simulink model "gm_sampleModel1618_sub"  (R2023a)
settings: Solver=VariableStepAuto  StartTime=0.0  StopTime=10.0  RelTol=1e-3
libraries: simulink x3, hdlsllib x2
settings Model: Creator=user1  LastModifiedBy=user1
settings OptimizationCC: BlockReduction=off  ConditionallyExecuteInputs=off
settings DebuggingCC: InheritedTsInSrcMsg=none

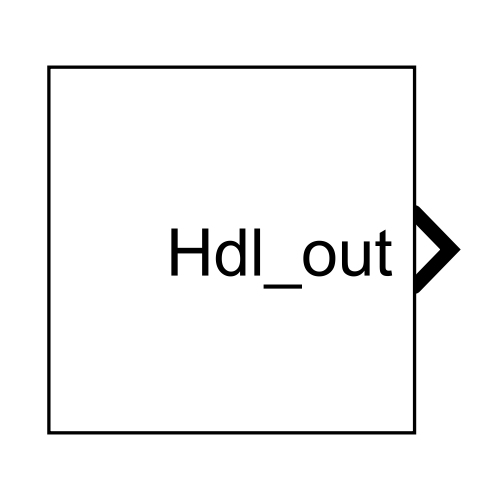
[thumbnail: Simulink's stored preview of the top-level diagram]
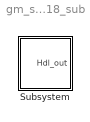
== system gm_sampleModel1618_sub ==
  Subsystem : Subsystem

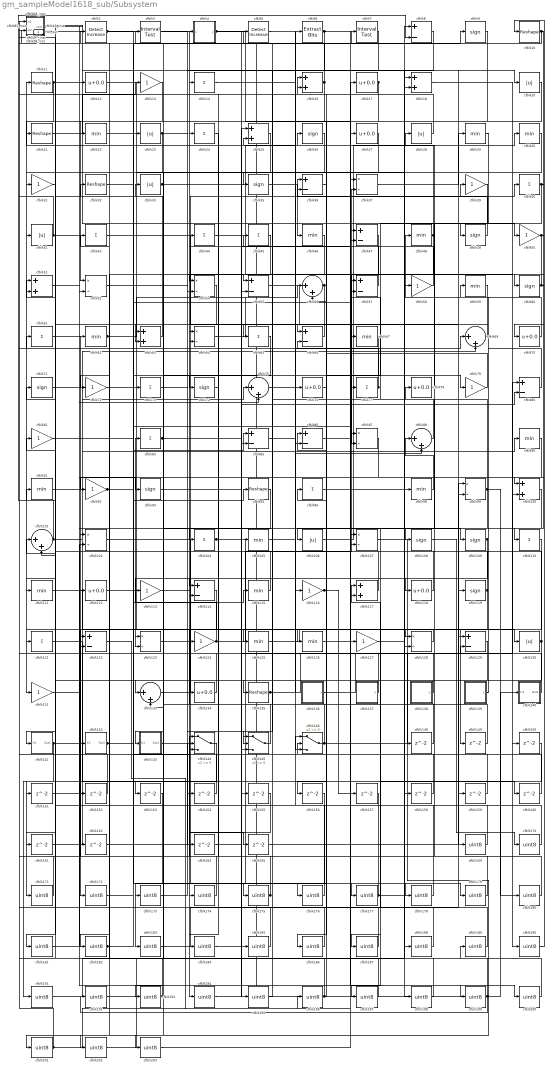
== system gm_sampleModel1618_sub/Subsystem ==
  cfblk1 : Constant  Value=0  OutDataTypeStr=uint8  SampleTime=1
  cfblk{10..11,21,32,95,135} (6 alike) : Reshape
  cfblk{16,18,25,51,63,100,117} (7 alike) : Sum  OutDataTypeStr=uint8
  cfblk{56,69,75,88,101,133} (6 alike) : Sum  Inputs=|++  OutDataTypeStr=uint8
  cfblk{37,52,54,64,87,99,102,107,123,128} (10 alike) : Product  Inputs=*/  OutDataTypeStr=uint8  RndMeth=Zero  SaturateOnIntegerOverflow=on
  cfblk{14,24,40,42,44..45,61,65,73,77,83,96,104,110,121} (15 alike) : Sum  Inputs=+  OutDataTypeStr=uint8
  cfblk{22,29..30,46,48,59,62,67,90..91,98,105,111,115,125..126} (16 alike) : MinMax  OutDataTypeStr=uint8
  cfblk{20,23,28,33,41,106,130} (7 alike) : Abs  OutDataTypeStr=uint8  SaturateOnIntegerOverflow=off
  cfblk{9,26,35,49,60,71,74,93,108..109,119} (11 alike) : Signum
  cfblk{12,17,27,70,76,78,112,118,134} (9 alike) : Bias  Bias=0.0  SaturateOnIntegerOverflow=off
  cfblk{13,31,39,50,58,72,79,81,92,113,116,124,127,131} (14 alike) : Gain  OutDataTypeStr=uint8
  cfblk{8,36,47,55,57,66,80,85..86,114,122,129} (12 alike) : Sum  Inputs=+-  OutDataTypeStr=uint8
  cfblk132_inst : Subsystem
  cfblk136 : Subsystem  mask(Counter Limited){uplimit=double(7), tsamp=double(-1)}
      mask prompts: uplimit "Simulink:masks:UpperLimit_MP"; tsamp "Simulink:masks:SampleTime_MP"
      mask help: Simulink:masks:CounterLimited_MD
      mask init:
      | nbits = double(8);
      | tsamp = double(-1);
      | uplimit = double(7);
  cfblk137 : Subsystem  mask(Counter Limited){uplimit=double(7), tsamp=double(-1)}
      mask prompts: uplimit "Simulink:masks:UpperLimit_MP"; tsamp "Simulink:masks:SampleTime_MP"
      mask help: Simulink:masks:CounterLimited_MD
      mask init:
      | nbits = double(8);
      | tsamp = double(-1);
      | uplimit = double(7);
  cfblk138 : Subsystem  mask(Counter Free-Running){NumBits=double(16), tsamp=double(-1)}
      mask prompts: NumBits "Simulink:masks:NumberOfBits_MP"; tsamp "Simulink:masks:SampleTime_MP"
      mask help: Simulink:masks:CounterFreeRunning_MD
  cfblk139 : Subsystem  mask(Counter Limited){uplimit=double(7), tsamp=double(-1)}
      mask prompts: uplimit "Simulink:masks:UpperLimit_MP"; tsamp "Simulink:masks:SampleTime_MP"
      mask help: Simulink:masks:CounterLimited_MD
      mask init:
      | nbits = double(8);
      | tsamp = double(-1);
      | uplimit = double(7);
  cfblk140 : Subsystem
  cfblk141 : Subsystem
  cfblk142 : Subsystem
  cfblk143 : Subsystem
  cfblk144 : Switch  OutDataTypeStr=uint8  SaturateOnIntegerOverflow=off  InputSameDT=off
  cfblk145 : Switch  OutDataTypeStr=uint8  SaturateOnIntegerOverflow=off  InputSameDT=off
  cfblk146 : Switch  OutDataTypeStr=uint8  SaturateOnIntegerOverflow=off  InputSameDT=off
  cfblk{148..162,164..165} (17 alike) : Delay  SampleTime=1
  cfblk15_inst : Subsystem
  cfblk{169..203} (35 alike) : DataTypeConversion  OutDataTypeStr=uint8  SaturateOnIntegerOverflow=off  RndMeth=Floor
  cfblk2 : simulink/Logic and Bit Operations/Detect Increase  vinit=0.0  OutDataTypeStr=uint8
      settings: LibrarySourceBlock=|
      | hdlsllib/Logic and Bit
      | Operations/Detect
      | Increase
  cfblk3 : hdlsllib/Logic and Bit Operations/Interval Test  IntervalClosedRight=on  uplimit=0.5  IntervalClosedLeft=on  lowlimit=-0.5  OutDataTypeStr=uint8
  cfblk34_inst : Subsystem
  cfblk38_inst : Subsystem
  cfblk4 : Subsystem  mask(Compare To Zero){relop=<=, OutDataTypeStr=uint8, ZeroCross=on}
      mask prompts: relop "Simulink:masks:Operator_MP"; OutDataTypeStr "Simulink:masks:OutputDataType_MP"; ZeroCross "Simulink:masks:EnableZerocrossingDetection_MP"
      mask help: Simulink:masks:CompareToZero_MD
      mask init:
      | OutDataTypeStr = 'uint8';
      | ZeroCross = 'on';
      | blkName = 'sampleModel1618_sub/Subsystem/cfblk4';
      | relop = '<=';
      | setValue = 'fixdt(0, 8)';
      mask TypeOptions relop: == | ~= | < | <= | >= | >
      mask TypeOptions OutDataTypeStr: Simulink:masks:uint8 | Simulink:masks:boolean
      mask Callback ZeroCross: sl('zeroCrossEnable', gcbh);
      mask Display: disp([relop,' 0'])
  cfblk43_inst : Subsystem
  cfblk5 : simulink/Logic and Bit Operations/Detect Increase  vinit=0.0  OutDataTypeStr=uint8
      settings: LibrarySourceBlock=|
      | hdlsllib/Logic and Bit
      | Operations/Detect
      | Increase
  cfblk6 : simulink/Logic and Bit Operations/Extract Bits  bitsToExtract=Upper half  numBits=8  bitIdxRange=[0 7]  outScalingMode=Preserve fixed-point scaling
      settings: LibrarySourceBlock=|
      | hdlsllib/Logic and Bit
      | Operations/Extract Bits
  cfblk68_inst : Subsystem
  cfblk7 : hdlsllib/Logic and Bit Operations/Interval Test  IntervalClosedRight=on  uplimit=0.5  IntervalClosedLeft=on  lowlimit=-0.5  OutDataTypeStr=uint8
  cfblk82_inst : Subsystem
  cfblk97_inst : Subsystem
  Hdl_out : Outport  OutDataTypeStr=uint8  SampleTime=1
  wires:
  cfblk1/1 -> cfblk50/1
  cfblk10/1 -> cfblk60/1, cfblk43_inst/2(in2)
  cfblk100/1 -> cfblk106/1
  cfblk101/1 -> cfblk8/2, cfblk109/1
  cfblk102/1 -> cfblk179/1
  cfblk104/1 -> cfblk178/1, cfblk105/1
  cfblk105/1 -> cfblk7/1
  cfblk106/1 -> cfblk30/1
  cfblk107/1 -> cfblk201/1
  cfblk108/1 -> cfblk170/1
  cfblk109/1 -> cfblk118/1, cfblk123/2
  cfblk11/1 -> cfblk12/1, cfblk131/1
  cfblk110/1 -> cfblk194/1
  cfblk111/1 -> cfblk130/1
  cfblk112/1 -> cfblk149/1
  cfblk113/1 -> cfblk175/1
  cfblk114/1 -> cfblk172/1
  cfblk115/1 -> cfblk61/1
  cfblk116/1 -> cfblk56/2, cfblk157/1, cfblk127/1
  cfblk117/1 -> cfblk71/1
  cfblk118/1 -> cfblk51/1
  cfblk119/1 -> cfblk38_inst/2(in2), cfblk143/1(In1)
  cfblk12/1 -> cfblk159/1
  cfblk121/1 -> cfblk153/1
  cfblk122/1 -> cfblk196/1
  cfblk123/1 -> cfblk4/1(u)
  cfblk124/1 -> cfblk37/2, cfblk83/1
  cfblk125/1 -> cfblk128/1
  cfblk126/1 -> cfblk37/1
  cfblk127/1 -> cfblk98/1
  cfblk128/1 -> cfblk121/1
  cfblk129/1 -> cfblk182/1
  cfblk13/1 -> cfblk52/1
  cfblk130/1 -> cfblk86/1, cfblk181/1
  cfblk131/1 -> cfblk62/1
  cfblk132_inst/1(out1) -> cfblk158/1
  cfblk133/1 -> cfblk39/1
  cfblk134/1 -> cfblk24/1
  cfblk135/1 -> cfblk76/1, cfblk99/1
  cfblk136/1(y) -> cfblk80/1
  cfblk137/1(y) -> cfblk132_inst/2(in2)
  cfblk138/1(y) -> cfblk8/1
  cfblk139/1(y) -> cfblk59/1
  cfblk14/1 -> cfblk116/1
  cfblk140/1(Out1) -> cfblk16/1
  cfblk141/1(Out1) -> cfblk191/1, cfblk90/1
  cfblk142/1(Out1) -> cfblk9/1, cfblk85/1
  cfblk143/1(Out1) -> cfblk165/1
  cfblk144/1 -> cfblk171/1
  cfblk145/1 -> cfblk97_inst/1(in1)
  cfblk146/1 -> cfblk100/2, cfblk64/1
  cfblk148/1 -> cfblk66/2
  cfblk149/1 -> cfblk114/2
  cfblk15_inst/1(out1) -> cfblk185/1
  cfblk150/1 -> cfblk197/1
  cfblk151/1 -> cfblk75/1
  cfblk152/1 -> cfblk51/2
  cfblk153/1 -> cfblk183/1
  cfblk154/1 -> cfblk101/1
  cfblk155/1 -> cfblk174/1
  cfblk156/1 -> cfblk173/1
  cfblk157/1 -> cfblk146/2
  cfblk158/1 -> cfblk64/2
  cfblk159/1 -> cfblk133/2
  cfblk16/1 -> cfblk135/1, cfblk3/1
  cfblk160/1 -> cfblk82_inst/1(in1)
  cfblk161/1 -> cfblk69/2
  cfblk162/1 -> cfblk195/1
  cfblk164/1 -> cfblk47/2
  cfblk165/1 -> cfblk119/1
  cfblk169/1 -> cfblk146/1
  cfblk17/1 -> cfblk85/2, cfblk156/1
  cfblk170/1 -> cfblk42/1
  cfblk171/1 -> cfblk82_inst/2(in2)
  cfblk172/1 -> cfblk144/1
  cfblk173/1 -> cfblk144/2
  cfblk174/1 -> cfblk144/3
  cfblk175/1 -> cfblk132_inst/1(in1), cfblk14/1
  cfblk176/1 -> cfblk113/1
  cfblk177/1 -> cfblk32/1, cfblk40/1
  cfblk178/1 -> cfblk81/1
  cfblk179/1 -> cfblk78/1
  cfblk18/1 -> cfblk190/1
  cfblk180/1 -> cfblk102/1
  cfblk181/1 -> cfblk102/2
  cfblk182/1 -> cfblk95/1, cfblk115/1
  cfblk183/1 -> cfblk129/1
  cfblk184/1 -> cfblk129/2
  cfblk185/1 -> cfblk152/1
  cfblk186/1 -> cfblk15_inst/1(in1)
  cfblk187/1 -> cfblk15_inst/2(in2)
  cfblk188/1 -> cfblk117/1
  cfblk189/1 -> cfblk96/1
  cfblk190/1 -> cfblk10/1
  cfblk191/1 -> cfblk18/1
  cfblk192/1 -> cfblk18/2
  cfblk193/1 -> cfblk43_inst/1(in1), cfblk142/1(In1)
  cfblk194/1 -> cfblk25/1
  cfblk195/1 -> cfblk25/2
  cfblk196/1 -> cfblk33/1, cfblk26/1
  cfblk197/1 -> cfblk122/1
  cfblk198/1 -> cfblk122/2
  cfblk199/1 -> cfblk192/1, cfblk189/1, Hdl_out/1, cfblk140/1(In1)
  cfblk2/1 -> cfblk86/2, cfblk125/1
  cfblk20/1 -> cfblk41/1
  cfblk200/1 -> cfblk91/1
  cfblk201/1 -> cfblk34_inst/1(in1), cfblk27/1
  cfblk202/1 -> cfblk107/1
  cfblk203/1 -> cfblk107/2
  cfblk21/1 -> cfblk13/1
  cfblk22/1 -> cfblk148/1
  cfblk23/1 -> cfblk55/1, cfblk31/1
  cfblk24/1 -> cfblk184/1
  cfblk25/1 -> cfblk193/1
  cfblk26/1 -> cfblk141/1(In1)
  cfblk27/1 -> cfblk114/1
  cfblk28/1 -> cfblk68_inst/1(in1)
  cfblk29/1 -> cfblk49/1
  cfblk3/1 -> cfblk145/2
  cfblk30/1 -> cfblk63/2
  cfblk31/1 -> cfblk111/1
  cfblk32/1 -> cfblk160/1
  cfblk33/1 -> cfblk6/1, cfblk87/2
  cfblk34_inst/1(out1) -> cfblk162/1
  cfblk35/1 -> cfblk46/1
  cfblk36/1 -> cfblk16/2
  cfblk37/1 -> cfblk29/1
  cfblk38_inst/1(out1) -> cfblk20/1, cfblk99/2
  cfblk39/1 -> cfblk108/1
  cfblk4/1(y) -> cfblk145/3, cfblk117/2
  cfblk40/1 -> cfblk70/1, cfblk67/1
  cfblk41/1 -> cfblk93/1, cfblk34_inst/2(in2)
  cfblk42/1 -> cfblk169/1
  cfblk43_inst/1(out1) -> cfblk52/2, cfblk73/1
  cfblk44/1 -> cfblk150/1
  cfblk45/1 -> cfblk72/1
  cfblk46/1 -> cfblk202/1
  cfblk47/1 -> cfblk55/2
  cfblk48/1 -> cfblk11/1, cfblk126/1
  cfblk49/1 -> cfblk36/1
  cfblk5/1 -> cfblk128/2
  cfblk50/1 -> cfblk146/3, cfblk110/1
  cfblk51/1 -> cfblk75/2
  cfblk52/1 -> cfblk134/1
  cfblk54/1 -> cfblk161/1
  cfblk55/1 -> cfblk198/1
  cfblk56/1 -> cfblk74/1, cfblk151/1
  cfblk57/1 -> cfblk44/1
  cfblk58/1 -> cfblk45/1
  cfblk59/1 -> cfblk77/1
  cfblk6/1 -> cfblk35/1, cfblk200/1
  cfblk60/1 -> cfblk100/1, cfblk54/1
  cfblk61/1 -> cfblk104/1
  cfblk62/1 -> cfblk56/1, cfblk79/1
  cfblk63/1 -> cfblk21/1
  cfblk64/1 -> cfblk47/1
  cfblk65/1 -> cfblk133/1
  cfblk66/1 -> cfblk63/1
  cfblk67/1 -> cfblk176/1
  cfblk68_inst/1(out1) -> cfblk154/1
  cfblk69/1 -> cfblk66/1
  cfblk7/1 -> cfblk54/2
  cfblk70/1 -> cfblk48/1
  cfblk71/1 -> cfblk112/1
  cfblk72/1 -> cfblk23/1
  cfblk73/1 -> cfblk164/1
  cfblk74/1 -> cfblk124/1
  cfblk75/1 -> cfblk69/1
  cfblk76/1 -> cfblk186/1
  cfblk77/1 -> cfblk97_inst/2(in2), cfblk68_inst/2(in2), cfblk38_inst/1(in1)
  cfblk78/1 -> cfblk28/1
  cfblk79/1 -> cfblk36/2
  cfblk8/1 -> cfblk145/1
  cfblk80/1 -> cfblk58/1
  cfblk81/1 -> cfblk177/1
  cfblk82_inst/1(out1) -> cfblk101/2
  cfblk83/1 -> cfblk87/1, cfblk155/1
  cfblk85/1 -> cfblk88/2
  cfblk86/1 -> cfblk17/1
  cfblk87/1 -> cfblk92/1
  cfblk88/1 -> cfblk57/1
  cfblk9/1 -> cfblk65/1
  cfblk90/1 -> cfblk203/1
  cfblk91/1 -> cfblk199/1
  cfblk92/1 -> cfblk57/2, cfblk2/1
  cfblk93/1 -> cfblk80/2
  cfblk95/1 -> cfblk123/1
  cfblk96/1 -> cfblk188/1
  cfblk97_inst/1(out1) -> cfblk22/1
  cfblk98/1 -> cfblk88/1
  cfblk99/1 -> cfblk187/1, cfblk180/1, cfblk5/1

== system gm_sampleModel1618_sub/Subsystem/cfblk132_inst ==
  in1 : Inport  OutDataTypeStr=uint8  SampleTime=1
  in2 : Inport  Port=2  OutDataTypeStr=uint8  SampleTime=1
  mul_cfblk132_dotp_mulcomp : Product  Inputs=**  OutDataTypeStr=uint8  SampleTime=1
  out1 : Outport  OutDataTypeStr=uint8  SampleTime=1
  wires:
  in1/1 -> mul_cfblk132_dotp_mulcomp/1
  in2/1 -> mul_cfblk132_dotp_mulcomp/2
  mul_cfblk132_dotp_mulcomp/1 -> out1/1

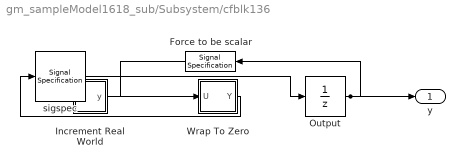
== system gm_sampleModel1618_sub/Subsystem/cfblk136 ==
  Force to be scalar : SignalSpecification  DisableCoverage=on  Dimensions=1
  Increment Real World : Subsystem  mask(Real World Value Increment){}
      mask help: Simulink:masks:RealWorldValueIncrement_MD
      mask Display: disp('V++')
  Output : UnitDelay  InitialCondition=0.0  SampleTime=tsamp  HasFrameUpgradeWarning=on
  Wrap To Zero : Subsystem  mask(Wrap To Zero){Threshold=double(7)}
      mask prompts: Threshold "Simulink:masks:Threshold_MP"
      mask help: Simulink:masks:WrapToZero_MD
  sigspec : SignalSpecification  OutDataTypeStr=uint8  Dimensions=1
  y : Outport  SampleTime=1
  wires:
  Force to be scalar/1 -> Increment Real World/1(u)
  Increment Real World/1(y) -> Wrap To Zero/1(U)
  Output/1 -> Force to be scalar/1, y/1
  Wrap To Zero/1(Y) -> sigspec/1
  sigspec/1 -> Output/1

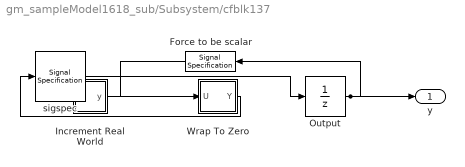
== system gm_sampleModel1618_sub/Subsystem/cfblk137 ==
  Force to be scalar : SignalSpecification  DisableCoverage=on  Dimensions=1
  Increment Real World : Subsystem  mask(Real World Value Increment){}
      mask help: Simulink:masks:RealWorldValueIncrement_MD
      mask Display: disp('V++')
  Output : UnitDelay  InitialCondition=0.0  SampleTime=tsamp  HasFrameUpgradeWarning=on
  Wrap To Zero : Subsystem  mask(Wrap To Zero){Threshold=double(7)}
      mask prompts: Threshold "Simulink:masks:Threshold_MP"
      mask help: Simulink:masks:WrapToZero_MD
  sigspec : SignalSpecification  OutDataTypeStr=uint8  Dimensions=1
  y : Outport  SampleTime=1
  wires:
  Force to be scalar/1 -> Increment Real World/1(u)
  Increment Real World/1(y) -> Wrap To Zero/1(U)
  Output/1 -> Force to be scalar/1, y/1
  Wrap To Zero/1(Y) -> sigspec/1
  sigspec/1 -> Output/1

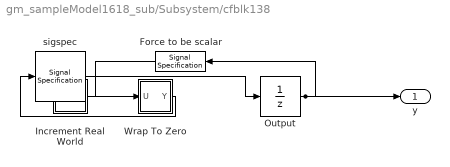
== system gm_sampleModel1618_sub/Subsystem/cfblk138 ==
  Force to be scalar : SignalSpecification  DisableCoverage=on  Dimensions=1
  Increment Real World : Subsystem  mask(Real World Value Increment){}
      mask help: Simulink:masks:RealWorldValueIncrement_MD
      mask Display: disp('V++')
  Output : UnitDelay  InitialCondition=0.0  SampleTime=tsamp  HasFrameUpgradeWarning=on
  Wrap To Zero : Subsystem  mask(Wrap To Zero){Threshold=double(65535)}
      mask prompts: Threshold "Simulink:masks:Threshold_MP"
      mask help: Simulink:masks:WrapToZero_MD
  sigspec : SignalSpecification  OutDataTypeStr=uint16  Dimensions=1
  y : Outport  SampleTime=1
  wires:
  Force to be scalar/1 -> Increment Real World/1(u)
  Increment Real World/1(y) -> Wrap To Zero/1(U)
  Output/1 -> Force to be scalar/1, y/1
  Wrap To Zero/1(Y) -> sigspec/1
  sigspec/1 -> Output/1

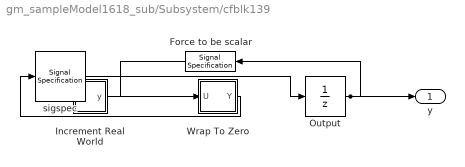
== system gm_sampleModel1618_sub/Subsystem/cfblk139 ==
  Force to be scalar : SignalSpecification  DisableCoverage=on  Dimensions=1
  Increment Real World : Subsystem  mask(Real World Value Increment){}
      mask help: Simulink:masks:RealWorldValueIncrement_MD
      mask Display: disp('V++')
  Output : UnitDelay  InitialCondition=0.0  SampleTime=tsamp  HasFrameUpgradeWarning=on
  Wrap To Zero : Subsystem  mask(Wrap To Zero){Threshold=double(7)}
      mask prompts: Threshold "Simulink:masks:Threshold_MP"
      mask help: Simulink:masks:WrapToZero_MD
  sigspec : SignalSpecification  OutDataTypeStr=uint8  Dimensions=1
  y : Outport  SampleTime=1
  wires:
  Force to be scalar/1 -> Increment Real World/1(u)
  Increment Real World/1(y) -> Wrap To Zero/1(U)
  Output/1 -> Force to be scalar/1, y/1
  Wrap To Zero/1(Y) -> sigspec/1
  sigspec/1 -> Output/1

== system gm_sampleModel1618_sub/Subsystem/cfblk140 ==
  In1 : Inport  OutDataTypeStr=uint8  PortDimensions=1  SampleTime=1
  Out1 : Outport  SampleTime=1
  wires:
  In1/1 -> Out1/1

== system gm_sampleModel1618_sub/Subsystem/cfblk141 ==
  In1 : Inport  OutDataTypeStr=uint8  PortDimensions=1  SampleTime=1
  Out1 : Outport  SampleTime=1
  wires:
  In1/1 -> Out1/1

== system gm_sampleModel1618_sub/Subsystem/cfblk142 ==
  In1 : Inport  OutDataTypeStr=uint8  PortDimensions=1  SampleTime=1
  Out1 : Outport  SampleTime=1
  wires:
  In1/1 -> Out1/1

== system gm_sampleModel1618_sub/Subsystem/cfblk143 ==
  In1 : Inport  OutDataTypeStr=uint8  PortDimensions=1  SampleTime=1
  Out1 : Outport  SampleTime=1
  wires:
  In1/1 -> Out1/1

== system gm_sampleModel1618_sub/Subsystem/cfblk15_inst ==
  in1 : Inport  OutDataTypeStr=uint8  SampleTime=1
  in2 : Inport  Port=2  OutDataTypeStr=uint8  SampleTime=1
  mul_cfblk15_dotp_mulcomp : Product  Inputs=**  OutDataTypeStr=uint8  SampleTime=1
  out1 : Outport  OutDataTypeStr=uint8  SampleTime=1
  wires:
  in1/1 -> mul_cfblk15_dotp_mulcomp/1
  in2/1 -> mul_cfblk15_dotp_mulcomp/2
  mul_cfblk15_dotp_mulcomp/1 -> out1/1

== system gm_sampleModel1618_sub/Subsystem/cfblk34_inst ==
  in1 : Inport  OutDataTypeStr=uint8  SampleTime=1
  in2 : Inport  Port=2  OutDataTypeStr=uint8  SampleTime=1
  mul_cfblk34_dotp_mulcomp : Product  Inputs=**  OutDataTypeStr=uint8  SampleTime=1
  out1 : Outport  OutDataTypeStr=uint8  SampleTime=1
  wires:
  in1/1 -> mul_cfblk34_dotp_mulcomp/1
  in2/1 -> mul_cfblk34_dotp_mulcomp/2
  mul_cfblk34_dotp_mulcomp/1 -> out1/1

== system gm_sampleModel1618_sub/Subsystem/cfblk38_inst ==
  in1 : Inport  OutDataTypeStr=uint8  SampleTime=1
  in2 : Inport  Port=2  OutDataTypeStr=uint8  SampleTime=1
  mul_cfblk38_dotp_mulcomp : Product  Inputs=**  OutDataTypeStr=uint8  SampleTime=1
  out1 : Outport  OutDataTypeStr=uint8  SampleTime=1
  wires:
  in1/1 -> mul_cfblk38_dotp_mulcomp/1
  in2/1 -> mul_cfblk38_dotp_mulcomp/2
  mul_cfblk38_dotp_mulcomp/1 -> out1/1

== system gm_sampleModel1618_sub/Subsystem/cfblk4 ==
  u : Inport  OutDataTypeStr=uint8  SampleTime=1
  Compare : RelationalOperator  Operator=<=  OutDataTypeStr=fixdt(0, 8)
  Constant : Constant  DisableCoverage=on  Value=0  OutDataTypeStr=Inherit: Inherit via back propagation  SampleTime=-1  PreserveConstantTs=on
  y : Outport  SampleTime=1
  wires:
  u/1 -> Compare/1
  Compare/1 -> y/1
  Constant/1 -> Compare/2

== system gm_sampleModel1618_sub/Subsystem/cfblk43_inst ==
  in1 : Inport  OutDataTypeStr=uint8  SampleTime=1
  in2 : Inport  Port=2  OutDataTypeStr=uint8  SampleTime=1
  mul_cfblk43_dotp_mulcomp : Product  Inputs=**  OutDataTypeStr=uint8  SampleTime=1
  out1 : Outport  OutDataTypeStr=uint8  SampleTime=1
  wires:
  in1/1 -> mul_cfblk43_dotp_mulcomp/1
  in2/1 -> mul_cfblk43_dotp_mulcomp/2
  mul_cfblk43_dotp_mulcomp/1 -> out1/1

== system gm_sampleModel1618_sub/Subsystem/cfblk68_inst ==
  in1 : Inport  OutDataTypeStr=uint8  SampleTime=1
  in2 : Inport  Port=2  OutDataTypeStr=uint8  SampleTime=1
  mul_cfblk68_dotp_mulcomp : Product  Inputs=**  OutDataTypeStr=uint8  SampleTime=1
  out1 : Outport  OutDataTypeStr=uint8  SampleTime=1
  wires:
  in1/1 -> mul_cfblk68_dotp_mulcomp/1
  in2/1 -> mul_cfblk68_dotp_mulcomp/2
  mul_cfblk68_dotp_mulcomp/1 -> out1/1

== system gm_sampleModel1618_sub/Subsystem/cfblk82_inst ==
  in1 : Inport  OutDataTypeStr=uint8  SampleTime=1
  in2 : Inport  Port=2  OutDataTypeStr=uint8  SampleTime=1
  mul_cfblk82_dotp_mulcomp : Product  Inputs=**  OutDataTypeStr=uint8  SampleTime=1
  out1 : Outport  OutDataTypeStr=uint8  SampleTime=1
  wires:
  in1/1 -> mul_cfblk82_dotp_mulcomp/1
  in2/1 -> mul_cfblk82_dotp_mulcomp/2
  mul_cfblk82_dotp_mulcomp/1 -> out1/1

== system gm_sampleModel1618_sub/Subsystem/cfblk97_inst ==
  in1 : Inport  OutDataTypeStr=uint8  SampleTime=1
  in2 : Inport  Port=2  OutDataTypeStr=uint8  SampleTime=1
  mul_cfblk97_dotp_mulcomp : Product  Inputs=**  OutDataTypeStr=uint8  SampleTime=1
  out1 : Outport  OutDataTypeStr=uint8  SampleTime=1
  wires:
  in1/1 -> mul_cfblk97_dotp_mulcomp/1
  in2/1 -> mul_cfblk97_dotp_mulcomp/2
  mul_cfblk97_dotp_mulcomp/1 -> out1/1

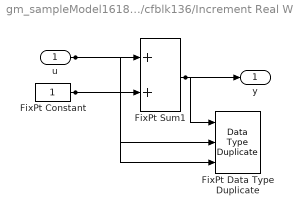
== system gm_sampleModel1618_sub/Subsystem/cfblk136/Increment Real World ==
  u : Inport  OutDataTypeStr=uint8  SampleTime=1
  FixPt Constant : Constant  DisableCoverage=on  OutDataTypeStr=Inherit: Inherit via back propagation  SampleTime=-1
  FixPt Data Type Duplicate : DataTypeDuplicate  DisableCoverage=on  NumInputPorts=3
  FixPt Sum1 : Sum  InputSameDT=on  OutDataTypeStr=Inherit: Inherit via back propagation  LockScale=on
  y : Outport  SampleTime=1
  wires:
  u/1 -> FixPt Sum1/1, FixPt Data Type Duplicate/2
  FixPt Constant/1 -> FixPt Sum1/2, FixPt Data Type Duplicate/3
  FixPt Sum1/1 -> FixPt Data Type Duplicate/1, y/1

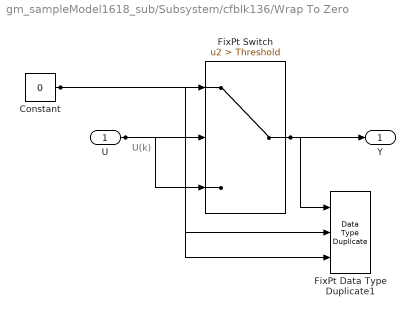
== system gm_sampleModel1618_sub/Subsystem/cfblk136/Wrap To Zero ==
  note: U(k)
  U : Inport  OutDataTypeStr=uint8  SampleTime=1
  Constant : Constant  DisableCoverage=on  Value=0  OutDataTypeStr=Inherit: Inherit via back propagation  SampleTime=-1
  FixPt Data Type Duplicate1 : DataTypeDuplicate  DisableCoverage=on  NumInputPorts=3
  FixPt Switch : Switch  Criteria=u2 > Threshold  Threshold=Threshold  OutDataTypeStr=Inherit: Inherit via back propagation  ZeroCross=off  SaturateOnIntegerOverflow=off  InputSameDT=off
  Y : Outport  SampleTime=1
  wires:
  U/1 -> FixPt Switch/3, FixPt Switch/2, FixPt Data Type Duplicate1/2
  Constant/1 -> FixPt Switch/1, FixPt Data Type Duplicate1/3
  FixPt Switch/1 -> FixPt Data Type Duplicate1/1, Y/1

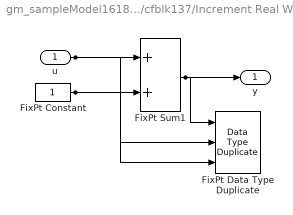
== system gm_sampleModel1618_sub/Subsystem/cfblk137/Increment Real World ==
  u : Inport  OutDataTypeStr=uint8  SampleTime=1
  FixPt Constant : Constant  DisableCoverage=on  OutDataTypeStr=Inherit: Inherit via back propagation  SampleTime=-1
  FixPt Data Type Duplicate : DataTypeDuplicate  DisableCoverage=on  NumInputPorts=3
  FixPt Sum1 : Sum  InputSameDT=on  OutDataTypeStr=Inherit: Inherit via back propagation  LockScale=on
  y : Outport  SampleTime=1
  wires:
  u/1 -> FixPt Sum1/1, FixPt Data Type Duplicate/2
  FixPt Constant/1 -> FixPt Sum1/2, FixPt Data Type Duplicate/3
  FixPt Sum1/1 -> FixPt Data Type Duplicate/1, y/1

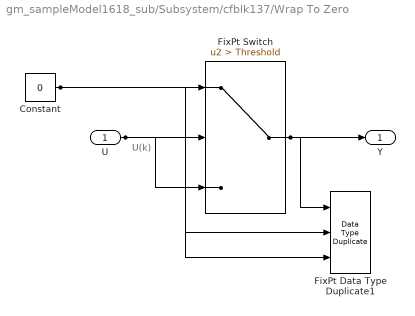
== system gm_sampleModel1618_sub/Subsystem/cfblk137/Wrap To Zero ==
  note: U(k)
  U : Inport  OutDataTypeStr=uint8  SampleTime=1
  Constant : Constant  DisableCoverage=on  Value=0  OutDataTypeStr=Inherit: Inherit via back propagation  SampleTime=-1
  FixPt Data Type Duplicate1 : DataTypeDuplicate  DisableCoverage=on  NumInputPorts=3
  FixPt Switch : Switch  Criteria=u2 > Threshold  Threshold=Threshold  OutDataTypeStr=Inherit: Inherit via back propagation  ZeroCross=off  SaturateOnIntegerOverflow=off  InputSameDT=off
  Y : Outport  SampleTime=1
  wires:
  U/1 -> FixPt Switch/3, FixPt Switch/2, FixPt Data Type Duplicate1/2
  Constant/1 -> FixPt Switch/1, FixPt Data Type Duplicate1/3
  FixPt Switch/1 -> FixPt Data Type Duplicate1/1, Y/1

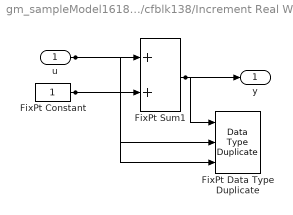
== system gm_sampleModel1618_sub/Subsystem/cfblk138/Increment Real World ==
  u : Inport  OutDataTypeStr=uint16  SampleTime=1
  FixPt Constant : Constant  DisableCoverage=on  OutDataTypeStr=Inherit: Inherit via back propagation  SampleTime=-1
  FixPt Data Type Duplicate : DataTypeDuplicate  DisableCoverage=on  NumInputPorts=3
  FixPt Sum1 : Sum  InputSameDT=on  OutDataTypeStr=Inherit: Inherit via back propagation  LockScale=on
  y : Outport  SampleTime=1
  wires:
  u/1 -> FixPt Sum1/1, FixPt Data Type Duplicate/2
  FixPt Constant/1 -> FixPt Sum1/2, FixPt Data Type Duplicate/3
  FixPt Sum1/1 -> FixPt Data Type Duplicate/1, y/1

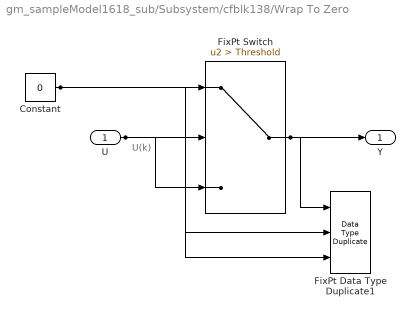
== system gm_sampleModel1618_sub/Subsystem/cfblk138/Wrap To Zero ==
  note: U(k)
  U : Inport  OutDataTypeStr=uint16  SampleTime=1
  Constant : Constant  DisableCoverage=on  Value=0  OutDataTypeStr=Inherit: Inherit via back propagation  SampleTime=-1
  FixPt Data Type Duplicate1 : DataTypeDuplicate  DisableCoverage=on  NumInputPorts=3
  FixPt Switch : Switch  Criteria=u2 > Threshold  Threshold=Threshold  OutDataTypeStr=Inherit: Inherit via back propagation  ZeroCross=off  SaturateOnIntegerOverflow=off  InputSameDT=off
  Y : Outport  SampleTime=1
  wires:
  U/1 -> FixPt Switch/3, FixPt Switch/2, FixPt Data Type Duplicate1/2
  Constant/1 -> FixPt Switch/1, FixPt Data Type Duplicate1/3
  FixPt Switch/1 -> FixPt Data Type Duplicate1/1, Y/1

== system gm_sampleModel1618_sub/Subsystem/cfblk139/Increment Real World ==
  u : Inport  OutDataTypeStr=uint8  SampleTime=1
  FixPt Constant : Constant  DisableCoverage=on  OutDataTypeStr=Inherit: Inherit via back propagation  SampleTime=-1
  FixPt Data Type Duplicate : DataTypeDuplicate  DisableCoverage=on  NumInputPorts=3
  FixPt Sum1 : Sum  InputSameDT=on  OutDataTypeStr=Inherit: Inherit via back propagation  LockScale=on
  y : Outport  SampleTime=1
  wires:
  u/1 -> FixPt Sum1/1, FixPt Data Type Duplicate/2
  FixPt Constant/1 -> FixPt Sum1/2, FixPt Data Type Duplicate/3
  FixPt Sum1/1 -> FixPt Data Type Duplicate/1, y/1

== system gm_sampleModel1618_sub/Subsystem/cfblk139/Wrap To Zero ==
  note: U(k)
  U : Inport  OutDataTypeStr=uint8  SampleTime=1
  Constant : Constant  DisableCoverage=on  Value=0  OutDataTypeStr=Inherit: Inherit via back propagation  SampleTime=-1
  FixPt Data Type Duplicate1 : DataTypeDuplicate  DisableCoverage=on  NumInputPorts=3
  FixPt Switch : Switch  Criteria=u2 > Threshold  Threshold=Threshold  OutDataTypeStr=Inherit: Inherit via back propagation  ZeroCross=off  SaturateOnIntegerOverflow=off  InputSameDT=off
  Y : Outport  SampleTime=1
  wires:
  U/1 -> FixPt Switch/3, FixPt Switch/2, FixPt Data Type Duplicate1/2
  Constant/1 -> FixPt Switch/1, FixPt Data Type Duplicate1/3
  FixPt Switch/1 -> FixPt Data Type Duplicate1/1, Y/1
